simulink model "HW6"  (R2018b)
settings: Solver=VariableStepAuto  StartTime=0.0  StopTime=10.0  RelTol=1e-3
undefined symbols (not defined in the file): a1, b1
settings Model: Creator=Raya  LastModifiedBy=Raya

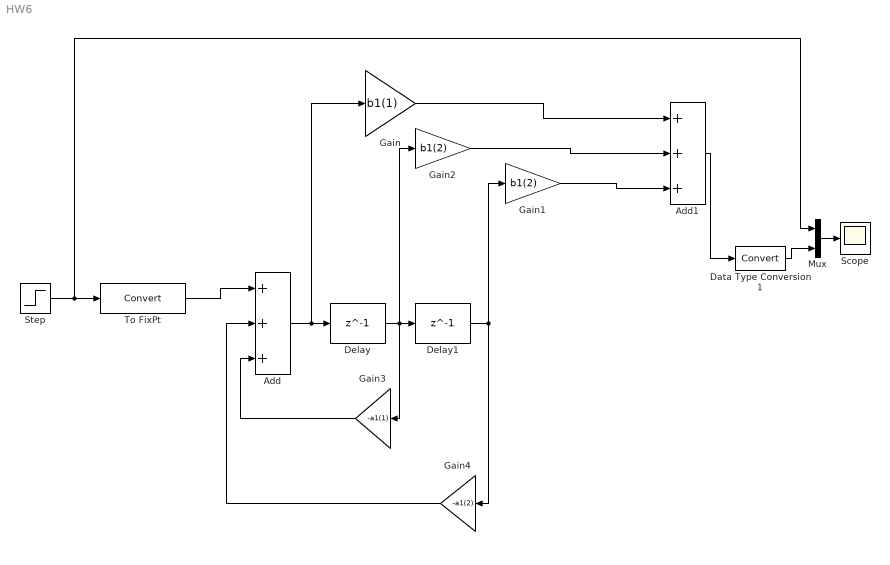
== system HW6 ==
  Add : Sum  Inputs=+++
  Add1 : Sum  Inputs=+++
  Data Type Conversion1 : DataTypeConversion
  Delay : Delay  DelayLength=1  InitialCondition=0  UseCircularBuffer=on
  Delay1 : Delay  DelayLength=1  InitialCondition=0  UseCircularBuffer=on
  Gain : Gain  Gain=b1(1)
  Gain1 : Gain  Gain=b1(2)
  Gain2 : Gain  Gain=b1(2)
  Gain3 : Gain  Gain=-a1(1)
  Gain4 : Gain  Gain=-a1(2)
  Mux : Mux  Inputs=2
  Scope : Scope
  Step : Step  SampleTime=0.001
  To FixPt : DataTypeConversion
  wires:
  Gain/1 -> Add1/1
  Gain2/1 -> Add1/2
  Gain1/1 -> Add1/3
  Delay1/1 -> Gain4/1, Gain1/1
  Delay/1 -> Gain2/1, Delay1/1, Gain3/1
  Add/1 -> Gain/1, Delay/1
  Data Type Conversion1/1 -> Mux/2
  Step/1 -> Mux/1, To FixPt/1
  Add1/1 -> Data Type Conversion1/1
  Mux/1 -> Scope/1
  Gain3/1 -> Add/3
  Gain4/1 -> Add/2
  To FixPt/1 -> Add/1
